simulink model "fullbridge"  (R2016a)
settings: Solver=ode4  StartTime=0.0  StopTime=0.1  FixedStep=1e-6  RelTol=1e-3
undefined symbols (not defined in the file): f_sw
libraries: dspsigops x2
settings Model: Creator=Heath  LastModifiedBy=Seth Barger
settings DataIOCC: LimitDataPoints=on  SaveFormat=Array  SignalLoggingSaveFormat=ModelDataLogs  SignalLoggingName=sigsOut
settings OptimizationCC: ExpressionDepthLimit=2147483647
settings DebuggingCC: SaveWithParameterizedLinksMsg=none  UnderspecifiedInitializationDetection=Classic  MergeDetectMultiDrivingBlocksExec=none  SignalResolutionControl=TryResolveAllWithWarning  MultiTaskDSMMsg=warning  MultiTaskCondExecSysMsg=none  StateNameClashWarn=warning  StrictBusMsg=None
settings HardwareCC: ProdBitPerPointer=32  ProdLargestAtomicFloat=None  ProdIntDivRoundTo=Undefined  ProdEndianess=Unspecified  ProdWordSize=32  ProdHWDeviceType=32-bit Generic  TargetUnknown=on
settings ModelReferenceCC: PropagateSignalLabelsOutOfModel=off
settings GRTTargetCC: CombineOutputUpdateFcns=off  GRTInterface=on
settings ConfigComp: CovModelRefEnable=Off

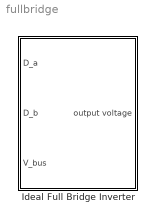
== system fullbridge ==
  "Ideal Full Bridge Inverter " : Subsystem

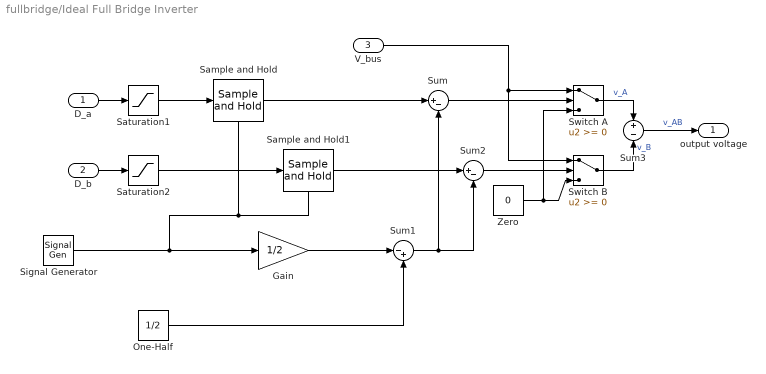
== system fullbridge/Ideal Full Bridge Inverter  ==
  D_a : Inport
  D_b : Inport  Port=2
  V_bus : Inport  Port=3
  Gain : Gain  Gain=1/2  SaturateOnIntegerOverflow=on  OutDataTypeStr=Inherit: Same as input  ParamDataTypeStr=Inherit: Same as input
  One-Half : Constant  Value=1/2
  Sample and Hold : dspsigops/Sample and Hold  trig=Falling edge  initCond=0  latchinput=off
  Sample and Hold1 : dspsigops/Sample and Hold  trig=Falling edge  initCond=0  latchinput=off
  Saturation1 : Saturate  UpperLimit=1  LowerLimit=0
  Saturation2 : Saturate  UpperLimit=1  LowerLimit=0
  Signal Generator : SignalGenerator  WaveForm=sawtooth  Frequency=f_sw
  Sum : Sum  Inputs=|+-  SaturateOnIntegerOverflow=on
  Sum1 : Sum  Inputs=|-+  SaturateOnIntegerOverflow=on
  Sum2 : Sum  Inputs=|+-  SaturateOnIntegerOverflow=on
  Sum3 : Sum  Inputs=+-  SaturateOnIntegerOverflow=on
  Switch A : Switch  SaturateOnIntegerOverflow=on
  Switch B : Switch  SaturateOnIntegerOverflow=on
  Zero : Constant  Value=0
  output voltage : Outport
  wires:
  Sum/1 -> Switch A/2
  Zero/1 -> Switch A/3, Switch B/3
  Signal Generator/1 -> Sample and Hold/Trigger, Sample and Hold1/Trigger, Gain/1
  Gain/1 -> Sum1/1
  One-Half/1 -> Sum1/2
  Sum2/1 -> Switch B/2
  Switch A/1 -> Sum3/1  "v_A"
  Switch B/1 -> Sum3/2  "v_B"
  Sum3/1 -> output voltage/1  "v_AB"
  Sum1/1 -> Sum2/2, Sum/2
  V_bus/1 -> Switch A/1, Switch B/1
  D_a/1 -> Saturation1/1
  Sample and Hold/1 -> Sum/1
  D_b/1 -> Saturation2/1
  Sample and Hold1/1 -> Sum2/1
  Saturation1/1 -> Sample and Hold/1
  Saturation2/1 -> Sample and Hold1/1
